simulink model "exp4_23"  (R2024b)
settings: Solver=VariableStepAuto  StartTime=0.0  StopTime=10  RelTol=1e-3
settings Model: Creator=86195  LastModifiedBy=86195

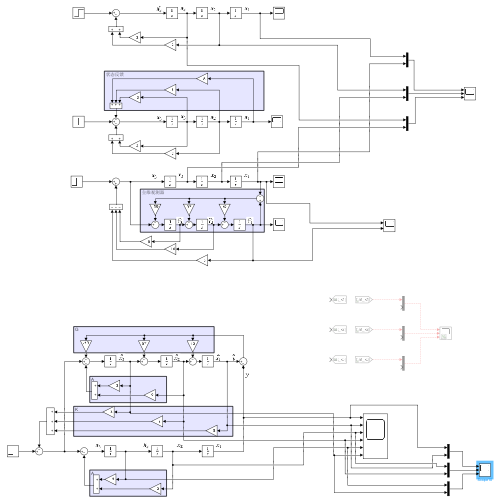
[thumbnail: Simulink's stored preview of the top-level diagram]
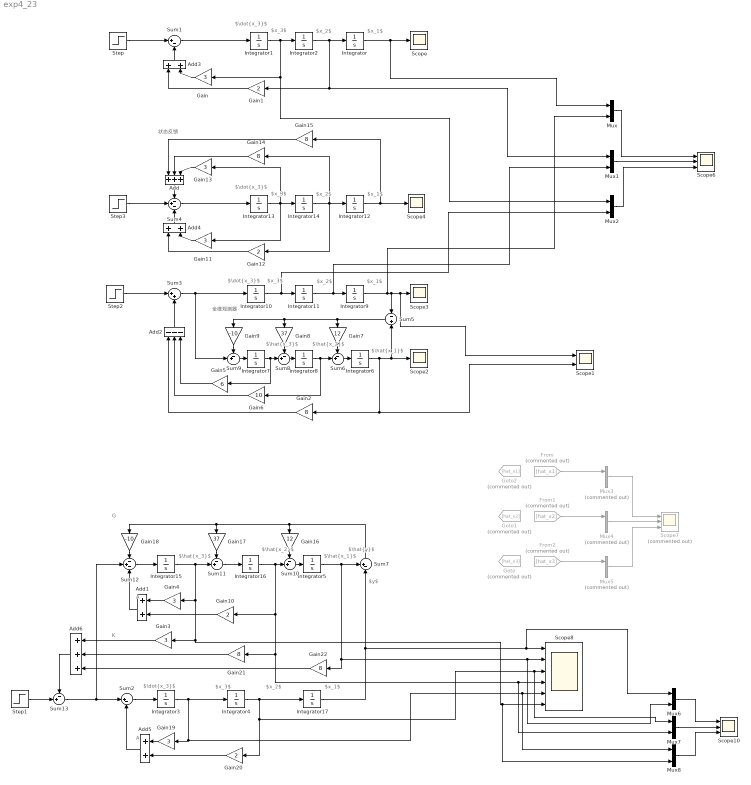
== system exp4_23 ==
  note: A
  note: 状态反馈
  note: $\hat{x_1}$
  note: $x_1$
  note: $x_2$
  note: $\dot{x_3}$
  note: $x_3$
  note: $\hat{x_2}$
  note: $\hat{x_3}$
  note: $x_1$
  note: $x_3$
  note: $\dot{x_3}$
  note: $x_2$
  note: $\dot{x_3}$
  note: $x_3$
  note: $x_1$
  note: $x_2$
  note: 全维观测器
  note: $x_2$
  note: $x_1$
  note: $x_3$
  note: $\dot{x_3}$
  note: $\hat{x_2}$
  note: $\hat{x_3}$
  note: $\hat{x_1}$
  note: $\hat{y}$
  note: $y$
  note: A
  note: G
  note: K
  Add : Sum  Inputs=+++
  Add{1,3..5} (4 alike) : Sum
  Add2 : Sum  Inputs=---
  Add6 : Sum  Inputs=+++
  From : From  Commented=on  GotoTag=hat_x1
  From1 : From  Commented=on  GotoTag=hat_x2
  From2 : From  Commented=on  GotoTag=hat_x3
  Gain{,3..4,11,13,19} (6 alike) : Gain  Gain=3
  Gain{1,10,12,20} (4 alike) : Gain  Gain=2
  Gain{2,14..15,21..22} (5 alike) : Gain  Gain=8
  Gain16 : Gain  Gain=12
  Gain17 : Gain  Gain=37
  Gain18 : Gain  Gain=-10
  Gain5 : Gain  Gain=6
  Gain6 : Gain  Gain=10
  Gain7 : Gain  Gain=12
  Gain8 : Gain  Gain=37
  Gain9 : Gain  Gain=-10
  Goto : Goto  Commented=on  GotoTag=hat_x3
  Goto1 : Goto  Commented=on  GotoTag=hat_x2
  Goto2 : Goto  Commented=on  GotoTag=hat_x1
  Integrator{,1..17} (18 alike) : Integrator
  Mux{,1..2,6..8} (6 alike) : Mux  Inputs=2
  Mux3 : Mux  Commented=on  Inputs=2
  Mux4 : Mux  Commented=on  Inputs=2
  Mux5 : Mux  Commented=on  Inputs=2
  Scope{,2..4} (4 alike) : Scope
  Scope1 : Scope  NumInputPorts=2
  Scope10 : Scope  NumInputPorts=3
  Scope6 : Scope  NumInputPorts=3
  Scope7 : Scope  Commented=on  NumInputPorts=3
  Scope8 : Scope  NumInputPorts=6
  Step{,1..3} (4 alike) : Step  SampleTime=0
  Sum1 : Sum  Inputs=|+-
  Sum{6,8..11,13} (6 alike) : Sum  Inputs=-+|
  Sum12 : Sum  Inputs=-+-
  Sum2 : Sum  Inputs=|+-
  Sum3 : Sum  Inputs=|++
  Sum4 : Sum  Inputs=-+-
  Sum5 : Sum  Inputs=-|+
  Sum7 : Sum  Inputs=+-|
  wires:
  Integrator2/1 -> Mux1/1, Gain1/1, Integrator/1
  Integrator/1 -> Mux/1, Scope/1
  Integrator1/1 -> Integrator2/1, Mux2/1, Gain/1
  Integrator6/1 -> Scope2/1, Sum5/2, Gain2/1, Scope1/2
  Integrator8/1 -> Sum6/2, Gain6/1
  Integrator7/1 -> Gain5/1, Sum8/2
  Integrator10/1 -> Mux2/2, Integrator11/1
  Integrator11/1 -> Mux1/2, Integrator9/1
  Integrator9/1 -> Mux/2, Scope1/1, Scope3/1, Sum5/1
  Sum6/1 -> Integrator6/1
  Gain7/1 -> Sum6/1
  Sum8/1 -> Integrator8/1
  Gain8/1 -> Sum8/1
  Sum9/1 -> Integrator7/1
  Gain9/1 -> Sum9/1
  Sum3/1 -> Integrator10/1, Sum9/2
  Step2/1 -> Sum3/1
  Sum5/1 -> Gain8/1, Gain9/1, Gain7/1
  Gain6/1 -> Add2/2
  Add2/1 -> Sum3/2
  Step/1 -> Sum1/1
  Sum1/1 -> Integrator1/1
  Add3/1 -> Sum1/2
  Gain/1 -> Add3/2
  Gain1/1 -> Add3/1
  Gain11/1 -> Add4/2
  Sum4/1 -> Integrator13/1
  Gain12/1 -> Add4/1
  Integrator14/1 -> Gain14/1, Gain12/1, Integrator12/1
  Integrator13/1 -> Gain13/1, Gain11/1, Integrator14/1
  Integrator12/1 -> Gain15/1, Scope4/1
  Step3/1 -> Sum4/2
  Add4/1 -> Sum4/3
  Add/1 -> Sum4/1
  Gain13/1 -> Add/3
  Gain14/1 -> Add/2
  Gain15/1 -> Add/1
  Gain5/1 -> Add2/3
  Gain2/1 -> Add2/1
  Mux/1 -> Scope6/1
  Mux1/1 -> Scope6/2
  Mux2/1 -> Scope6/3
  Integrator4/1 -> Integrator17/1, Mux7/1, Scope8/3, Gain20/1
  Integrator17/1 -> Mux6/1, Scope8/1, Sum7/2
  Sum2/1 -> Integrator3/1
  Integrator3/1 -> Integrator4/1, Mux8/1, Scope8/5, Gain19/1
  Step1/1 -> Sum13/2
  Add1/1 -> Sum12/3
  Integrator15/1 -> Sum11/2, Gain4/1, Mux8/2, Scope8/6, Gain3/1
  Integrator16/1 -> Sum10/2, Mux7/2, Scope8/4, Gain21/1, Gain10/1
  Gain16/1 -> Sum10/1
  Sum11/1 -> Integrator16/1
  Sum10/1 -> Integrator5/1
  Gain17/1 -> Sum11/1
  Sum12/1 -> Integrator15/1
  Gain18/1 -> Sum12/1
  Sum7/1 -> Gain18/1, Gain17/1, Gain16/1
  Integrator5/1 -> Sum7/1, Mux6/2, Scope8/2, Gain22/1
  Add6/1 -> Sum13/1
  Gain22/1 -> Add6/3
  Sum13/1 -> Sum2/1, Sum12/2
  Add5/1 -> Sum2/2
  Gain19/1 -> Add5/1
  Gain20/1 -> Add5/2
  Gain21/1 -> Add6/2
  Gain3/1 -> Add6/1
  Gain4/1 -> Add1/1
  Gain10/1 -> Add1/2
  Mux3/1 -> Scope7/1
  Mux4/1 -> Scope7/2
  Mux5/1 -> Scope7/3
  From/1 -> Mux3/1
  From1/1 -> Mux4/1
  From2/1 -> Mux5/1
  Mux6/1 -> Scope10/1
  Mux7/1 -> Scope10/2
  Mux8/1 -> Scope10/3
